simulink model "pacejka_longitudinal_model"  (R2018b)
settings: Solver=FixedStepAuto  StartTime=0.0  StopTime=10.0  FixedStep=0.01  RelTol=1e-3
undefined symbols (not defined in the file or in its folder): a1, a2, B, C
settings Model: Creator=Cassio.Freitas  LastModifiedBy=Cassio.Freitas

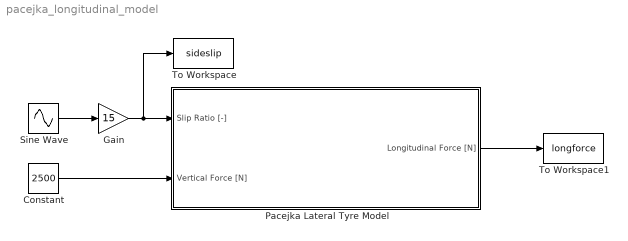
== system pacejka_longitudinal_model ==
  Constant : Constant  Value=2500
  Gain : Gain  Gain=15
  Pacejka Lateral Tyre Model : Subsystem
  Sine Wave : Sin  SampleTime=0
  To Workspace : ToWorkspace  VariableName=sideslip  SaveFormat=Timeseries  SampleTime=-1
  To Workspace1 : ToWorkspace  VariableName=longforce  SaveFormat=Timeseries  SampleTime=-1
  wires:
  Constant/1 -> Pacejka Lateral Tyre Model/2(Vertical Force [N])
  Sine Wave/1 -> Gain/1
  Gain/1 -> To Workspace/1, Pacejka Lateral Tyre Model/1(Slip Ratio [-])
  Pacejka Lateral Tyre Model/1(Longitudinal Force [N]) -> To Workspace1/1

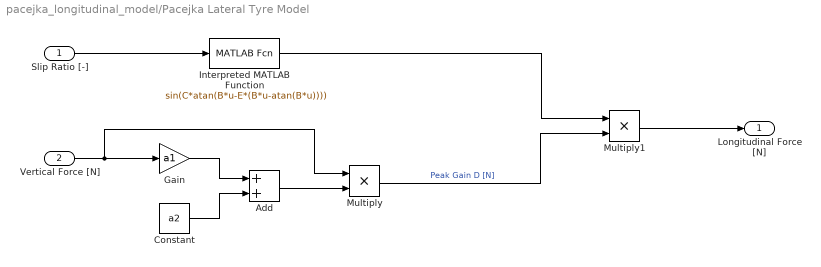
== system pacejka_longitudinal_model/Pacejka Lateral Tyre Model ==
  Slip Ratio [-] : Inport
  Vertical Force [N] : Inport  Port=2
  Add : Sum
  Constant : Constant  Value=a2
  Gain : Gain  Gain=a1
  Interpreted MATLAB Function : MATLABFcn  MATLABFcn=sin(C*atan(B*u-E*(B*u-atan(B*u))))
  Multiply : Product
  Multiply1 : Product
  Longitudinal Force [N] : Outport
  wires:
  Vertical Force [N]/1 -> Multiply/1, Gain/1
  Constant/1 -> Add/2
  Gain/1 -> Add/1
  Add/1 -> Multiply/2
  Multiply/1 -> Multiply1/2  "Peak Gain D [N]"
  Slip Ratio [-]/1 -> Interpreted MATLAB Function/1
  Interpreted MATLAB Function/1 -> Multiply1/1
  Multiply1/1 -> Longitudinal Force [N]/1
